simulink model "dev_blk"  (Simulink 7.8)
settings: Solver=ode45  StartTime=0.0  StopTime=10.0  RelTol=1e-3
settings Model: Creator=MD710  LastModifiedBy=MD710

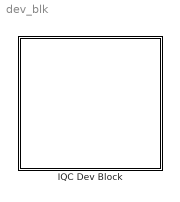
== system dev_blk ==
  IQC Dev Block : Subsystem
      mask Display: disp('IQC Dev Block')

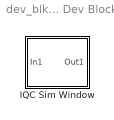
== system dev_blk/IQC Dev Block ==
  IQC Sim Window : Subsystem  mask(IQC Sim Window(ver:0.1)){sou_del=Random, max_del=10, num_ran=1, cus=1, var_nam='', iqc1=on, iqc1_pole=[], iqc1_out='', iqc2=off, lis_rel='', delay_time=0}
      mask prompts: sou_del "Source of the delay:(Default: Random)"; max_del "Maximum Delay:"; num_ran "The Number of Random:(1 or input_dim)"; cus "Custom:"; var_nam "Variable Name:(Default: empty)"; iqc1 "iqc_window(Input,Maximum Delay,Pole)"; iqc1_pole "Pole:(Default: [])"; iqc1_out "Output Variable:(Default: empty)"; iqc2 "Custom IQC"; lis_rel "List of IQC Relationships:"
      mask init:
      | switch sou_del
      |     case 1
      |         delay_time=max_del*rand(1,num_ran);
      |     case 2
      |         delay_time=reshape(cus,1,length(cus));
      | end
      mask Help: <a href="matlab:doc iqc_window;">iqc_window</a>
      mask StyleString: popup(Random|Custom),edit,edit,edit,edit,checkbox,edit,edit,checkbox,edit,edit
      mask CallbackString: iqc_block_cho(gcb,'sim_window_sou')|||||iqc_block_cho(gcb,'sim_window_iqc1')|||iqc_block_cho(gcb,'sim_window_iqc2')||
      mask TabNameString: Simulink Parameters,Simulink Parameters,Simulink Parameters,Simulink Parameters,Simulink Parameters,Procedure Parameters,Procedure Parameters,Procedure Parameters,Procedure Parameters,Procedure Parameters,Simulink Parameters
      mask Display:
      | text(5,85,'Sim IQC')
      | plot(0,0,100,100,[84,94,4],[27,25,25],[94,84],[25,22],[15,15],[5,97],[12,15],[86,97],[18,15],[86,97],[81,70,70,16,16,6],[26,26,72,72,26,26],[71,71,15],[26,73,73])

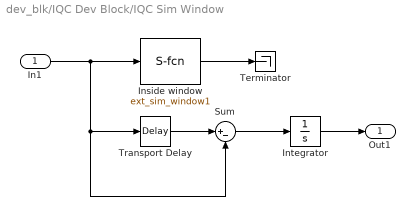
== system dev_blk/IQC Dev Block/IQC Sim Window ==
  In1 : Inport
  Inside window : M-S-Function  FunctionName=ext_sim_window1  Parameters=sou_del,max_del,num_ran,cus,var_nam,iqc1,iqc1_pole,iqc1_out,iqc2,lis_rel,delay_time
  Integrator : Integrator
  Sum : Sum  Inputs=|+-
  Terminator : Terminator
  Transport Delay : TransportDelay  DelayTime=delay_time
  Out1 : Outport
  wires:
  In1/1 -> Inside window/1, Transport Delay/1, Sum/2
  Inside window/1 -> Terminator/1
  Transport Delay/1 -> Sum/1
  Sum/1 -> Integrator/1
  Integrator/1 -> Out1/1
